simulink model "a"  (R2018a)
settings: Solver=VariableStepAuto  StartTime=0.0  StopTime=100.0  RelTol=1e-3
undefined symbols (not defined in the file): K_c, K_r
libraries: cstblocks x1, simulink x1
settings Model: Creator=Ale  LastModifiedBy=Ale

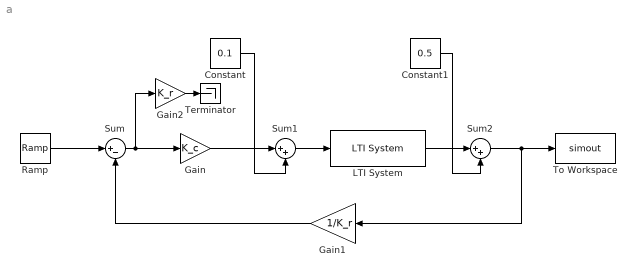
== system a ==
  Constant : Constant  Value=0.1
  Constant1 : Constant  Value=0.5
  Gain : Gain  Gain=K_c
  Gain1 : Gain  Gain=1/K_r
  Gain2 : Gain  Gain=K_r
  LTI System : cstblocks/LTI System  sys=F  IC=[]
  Ramp : simulink/Sources/Ramp  slope=1  start=0  InitialOutput=0
  Sum : Sum  Inputs=|+-
  Sum1 : Sum  Inputs=|++
  Sum2 : Sum  Inputs=|++
  Terminator : Terminator
  To Workspace : ToWorkspace  VariableName=simout  SaveFormat=Timeseries  SampleTime=-1
  wires:
  Ramp/1 -> Sum/1
  Sum/1 -> Gain2/1, Gain/1
  Gain/1 -> Sum1/1
  Constant/1 -> Sum1/2
  Constant1/1 -> Sum2/2
  Sum2/1 -> Gain1/1, To Workspace/1
  Gain1/1 -> Sum/2
  Gain2/1 -> Terminator/1
  Sum1/1 -> LTI System/1
  LTI System/1 -> Sum2/1
